simulink model "M1_regOBA_2020b"  (R2020b)
settings: Solver=VariableStepAuto  StartTime=0.0  StopTime=80  RelTol=1e-3
values from neighbouring files (symbols this model uses):
  fsz = 2500    [o01S_model_skryptdrugi.m]
  Jeq = JL + J    (= 3.228252e-05)    [o01S_model_skryptdrugi.m]
  K_windup_p = 1    [o01S_model_skryptdrugi.m]
  K_windup_v = 3    [o01S_model_skryptdrugi.m]
  Km = 0.0257    [o01S_model_skryptdrugi.m]
  Kp_p = 2    [o01S_model_skryptdrugi.m]
  Kp_v = 0.04604    [o01S_model_skryptdrugi.m]
  Psz = 0.005    [o01S_model_skryptdrugi.m]
  Rm = 2.675    [o01S_model_skryptdrugi.m]
  Td_p = 0    [o01S_model_skryptdrugi.m]
  Td_v = 0    [o01S_model_skryptdrugi.m]
  Ti_v = 0.17    [o01S_model_skryptdrugi.m]
  w_filtr_pom = 1/10    (= 0.1)    [o01S_model_skryptdrugi.m]
libraries: simulink x1
settings Model: Creator=Adam  LastModifiedBy=Adam
settings SolverCC: ZeroCrossAlgorithm=Adaptive
settings DebuggingCC: IgnoredZcDiagnostic=none

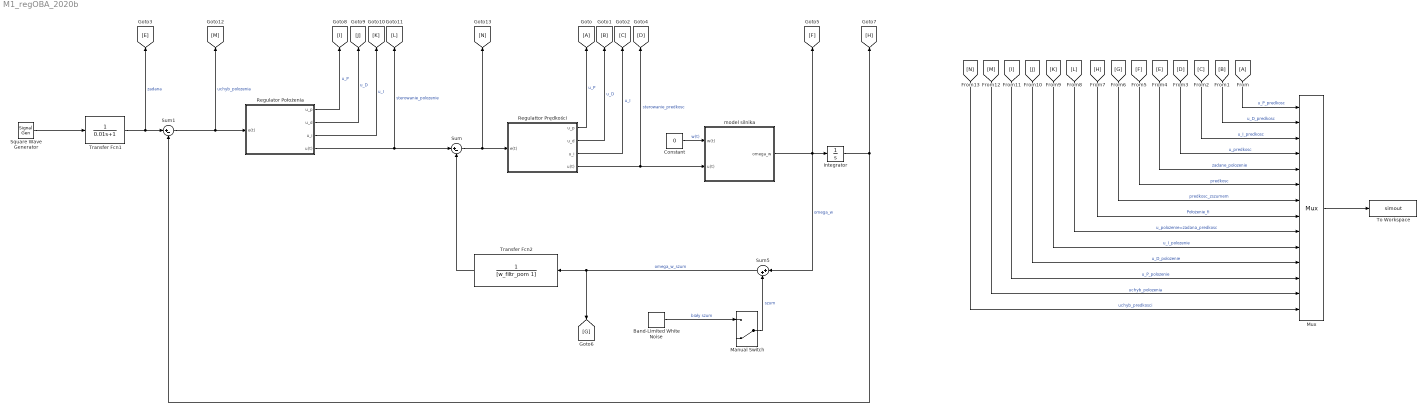
== system M1_regOBA_2020b ==
  Band-Limited White Noise : simulink/Sources/Band-Limited White Noise  Cov=[Psz]  Ts=0.1  seed=[fsz]
  Constant : Constant  Value=0
  Integrator : Integrator
  Manual Switch : ManualSwitch  CurrentSetting=0
  Mux : Mux  Inputs=14
  Regulator Położenia : Subsystem
  Regulattor Prędkości : Subsystem
  Square Wave Generator : SignalGenerator  WaveForm=square  Amplitude=9  Frequency=0.08
  Sum : Sum  Inputs=|+-
  Sum1 : Sum  Inputs=|+-
  Sum5 : Sum  Inputs=|++
  To Workspace : ToWorkspace  VariableName=simout  SaveFormat=Timeseries  SampleTime=-1
  Transfer Fcn1 : TransferFcn  Denominator=[0.01 1]
  Transfer Fcn2 : TransferFcn  Denominator=[w_filtr_pom 1]
  model silnika : Subsystem
  wires:
  Constant/1 -> model silnika/1(w(t))  "w(t)"
  model silnika/1(omega_w) -> Sum5/1, [F], Integrator/1  "omega_w"
  Regulattor Prędkości/4(u(t)) -> model silnika/2(u(t)), [D]  "sterowanie_predkosc"
  Regulattor Prędkości/1(u_p) -> [A]  "u_P"
  Regulattor Prędkości/3(u_i) -> [C]  "u_I"
  Regulattor Prędkości/2(u_d) -> [B]  "u_D"
  Integrator/1 -> [H], Sum1/2
  Manual Switch/1 -> Sum5/2  "szum"
  Sum5/1 -> Transfer Fcn2/1, [G]  "omega_w_szum"
  Band-Limited White Noise/1 -> Manual Switch/1  "biały szum"
  Transfer Fcn2/1 -> Sum/2
  Sum/1 -> Regulattor Prędkości/1(e(t)), [N]
  Square Wave Generator/1 -> Transfer Fcn1/1
  [F] -> Mux/6  "predkosc"
  [A] -> Mux/1  "u_P_predkosc"
  [K] -> Mux/10  "u_I_polozenie"
  [I] -> Mux/12  "u_P_polozenie"
  [N] -> Mux/14  "uchyb_predkosci"
  [G] -> Mux/7  "predkosc_zszumem"
  [M] -> Mux/13  "uchyb_polozenia"
  [L] -> Mux/9  "u_polozenie=zadana_predkosc"
  [J] -> Mux/11  "u_D_polozenie"
  [H] -> Mux/8  "Położenie_fi"
  [B] -> Mux/2  "u_D_predkosc"
  [D] -> Mux/4  "u_predkosc"
  [C] -> Mux/3  "u_I_predkosc"
  [E] -> Mux/5  "zadane_polozenie"
  Mux/1 -> To Workspace/1
  Regulator Położenia/4(u(t)) -> Sum/1, [L]  "sterowanie_polozenie"
  Regulator Położenia/2(u_d) -> [J]  "u_D"
  Regulator Położenia/1(u_p) -> [I]  "u_P"
  Sum1/1 -> [M], Regulator Położenia/1(e(t))  "uchyb_polozenia"
  Regulator Położenia/3(u_i) -> [K]  "u_I"
  Transfer Fcn1/1 -> Sum1/1, [E]  "zadana"

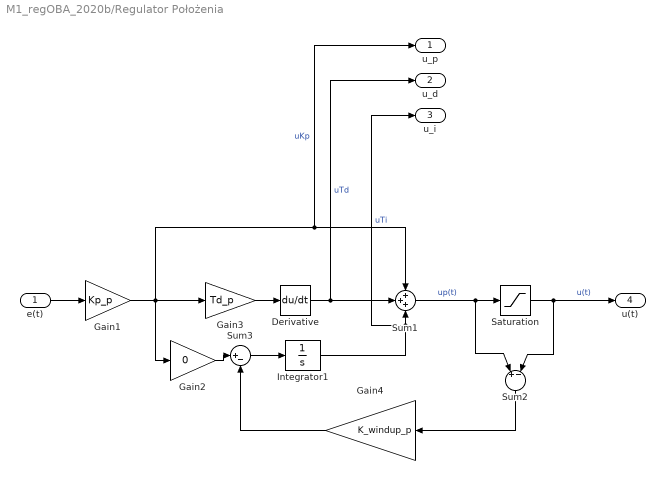
== system M1_regOBA_2020b/Regulator Położenia ==
  e(t) : Inport
  Derivative : Derivative  CoefficientInTFapproximation=500
  Gain1 : Gain  Gain=Kp_p
  Gain2 : Gain  Gain=0
  Gain3 : Gain  Gain=Td_p
  Gain4 : Gain  Gain=K_windup_p
  Integrator1 : Integrator
  Saturation : Saturate  UpperLimit=300  LowerLimit=-300  ZeroCross=off
  Sum1 : Sum  Inputs=+++
  Sum2 : Sum  Inputs=|+-|
  Sum3 : Sum  Inputs=|+-
  u_p : Outport
  u_d : Outport  Port=2
  u_i : Outport  Port=3
  u(t) : Outport  Port=4
  wires:
  Sum1/1 -> Saturation/1, Sum2/1  "up(t)"
  Gain2/1 -> Sum3/1
  Sum2/1 -> Gain4/1
  Gain4/1 -> Sum3/2
  Derivative/1 -> u_d/1, Sum1/2  "uTd"
  Gain3/1 -> Derivative/1
  Gain1/1 -> u_p/1, Sum1/1, Gain3/1, Gain2/1  "uKp"
  Integrator1/1 -> u_i/1, Sum1/3  "uTi"
  Sum3/1 -> Integrator1/1
  Saturation/1 -> u(t)/1, Sum2/2  "u(t)"
  e(t)/1 -> Gain1/1

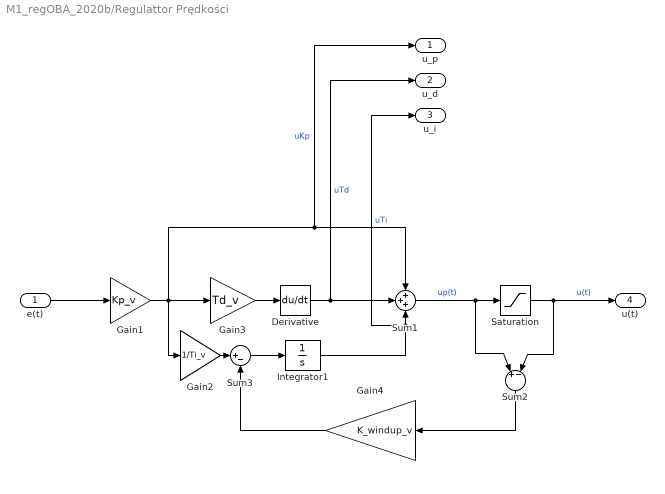
== system M1_regOBA_2020b/Regulattor Prędkości ==
  e(t) : Inport
  Derivative : Derivative  CoefficientInTFapproximation=500
  Gain1 : Gain  Gain=Kp_v
  Gain2 : Gain  Gain=1/Ti_v
  Gain3 : Gain  Gain=Td_v
  Gain4 : Gain  Gain=K_windup_v
  Integrator1 : Integrator
  Saturation : Saturate  UpperLimit=10  LowerLimit=-10  ZeroCross=off
  Sum1 : Sum  Inputs=+++
  Sum2 : Sum  Inputs=|+-|
  Sum3 : Sum  Inputs=|+-
  u_p : Outport
  u_d : Outport  Port=2
  u_i : Outport  Port=3
  u(t) : Outport  Port=4
  wires:
  Sum1/1 -> Saturation/1, Sum2/1  "up(t)"
  Gain2/1 -> Sum3/1
  Sum2/1 -> Gain4/1
  Gain4/1 -> Sum3/2
  Derivative/1 -> u_d/1, Sum1/2  "uTd"
  Gain3/1 -> Derivative/1
  Gain1/1 -> u_p/1, Sum1/1, Gain3/1, Gain2/1  "uKp"
  Integrator1/1 -> u_i/1, Sum1/3  "uTi"
  Sum3/1 -> Integrator1/1
  Saturation/1 -> u(t)/1, Sum2/2  "u(t)"
  e(t)/1 -> Gain1/1

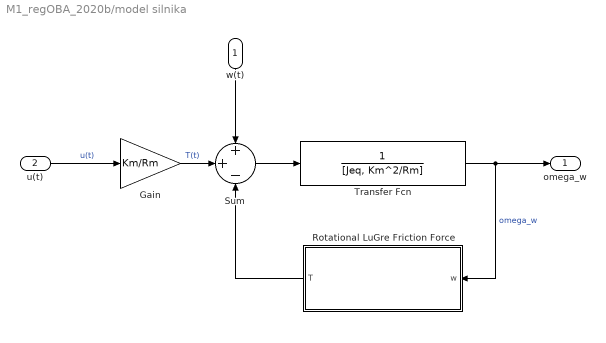
== system M1_regOBA_2020b/model silnika ==
  w(t) : Inport
  u(t) : Inport  Port=2
  Gain : Gain  Gain=Km/Rm
  Rotational LuGre Friction Force : Subsystem  TreatAsAtomicUnit=on  mask(LuGre friction model){ro0=1.2, ro1=0.05, ro2=2.9e-6, Fc=0.77e-3, Fs=12e-3, Vs=0.09}
      mask prompts: Fc "Culomb force (Fc)"; Fs "Friction force (Fs)"; Vs "Striback velocity (Vs)"
      mask help:
      | The LuGre model is a dynamic friction model. The model is related to the bristle interpretation of friction. Friction is modeled as the average deflection force of elastic springs. When a tangential force is applied the bristles will deflect like springs. If the deflection is sufficiently large the bristles start to slip.
      |
      | The input signal is the velocity of the object. The output signal is the fristion force value.
      mask Help:
      | <!DOCTYPE html   PUBLIC "-//W3C//DTD HTML 4.01 Transitional//EN" "http://www.w3.org/TR/1999/REC-html401-19991224/loose.dtd">
      | <html lang="en"><head>
      | <meta http-equiv="Content-Type" content="text/html; charset=utf-8">
      | <title>About :: LuGre friction model</title>
      | <meta name="description" content="">
      | </head>
      | <body><a name="top_of_page"></a>
      | The LuGre model is a dynamic friction model. The model is related to
      | the bristle interpretation of friction. Friction is modeled as the average
      | deflection force of elastic springs. When a tangential force is applied the bristles
      | will deflect like springs. If the deflection is sufficiently large the bristles start
      | to slip. The average bristle deflection for a steady state motion is determined
      | by the velocity. It is lower at low velocities, which implies that the steady state
      | deflection decreases with increasing velocity. This models the phenomenon that
      | the surfaces are pushed apart by the lubricant, and models the Stribeck effect.
      | The model also includes rate dependent friction phenomena such as varying
      | break-away force and frictional lag.<sup><a href="#ref1">1</a></sup></p><p>More information about the model may be found in the labsheets.</p>
      | <hr><small>
      | <sup><a name="ref1"></a>1</sup> <b>Friction Models and Friction Compensation</b>. H. Olsson, K.J. &Aring;str&ouml;m, C. Canudas de Wit, M. G&auml;fvert, P. Lischinsky
      | </small>
      | <br />
      | <br />
      | <hr>
      | <center><small>Copyright&copy;2009
      | <a href="mailto:w.kurek@ely.pg.gda.pl">Wojciech Kurek</a>,
      | <a href="mailto:g.ewald@ely.pg.gda.pl">Grzegorz Ewald</a>
      | </small></center>
      | </body>
      | </html>
      mask Callback ro0:
      | if str2num(get_param(gcb, 'ro0')) <= 0
      |     error('ro0 is negative!')
      | end
      mask Callback ro1:
      | if str2num(get_param(gcb, 'ro1')) <= 0
      |     error('ro1 is negative!')
      | end
      mask Callback ro2:
      | if str2num(get_param(gcb, 'ro2')) <= 0
      |     error('ro2 is negative!')
      | end
      mask Callback Fc:
      | if str2num(get_param(gcb, 'Fs')) <= 0
      |     error('Culomb force is negative!')
      | end
      mask Callback Fs:
      | if str2num(get_param(gcb, 'Fs')) <= 0
      |     error('Friction force is negative!')
      | end
      mask Callback Vs:
      | if str2num(get_param(gcb, 'Vs')) <= 0
      |     error('Striback velocity is negative!')
      | end
      mask Display:
      | patch([0.1 0.1 0.9 0.9],[0.1 0.25 0.25 0.1],[0.8 0.8 0.8])
      | patch([0.1 0.1 0.9 0.9],[0.9 0.75 0.75 0.9],[0.8 0.8 0.8])
      | 
      | plot([0.12 0.12],[0.25 0.5])
      | plot([0.2 0.2],[0.25 0.5])
      | plot([0.4 0.4],[0.25 0.5])
      | plot([0.57 0.57],[0.25 0.5])
      | plot([0.67 0.67],[0.25 0.5])
      | plot([0.87 0.87],[0.25 0.5])
      | 
      | plot([0.17 0.18 0.2 0.23],[0.75 0.6 0.5 0.45])
      | plot([0.35 0.36 0.39 0.44],[0.75 0.6 0.5 0.48])
      | plot([0.62 0.64 0.68 0.72],[0.75 0.6 0.5 0.48])
      | plot([0.85 0.86 0.87 0.89],[0.75 0.6 0.5 0.48])
      | 
      | plot([0.15 0.15],[0.75 0.4])
      | plot([0.28 0.28],[0.75 0.4])
      | plot([0.55 0.55],[0.75 0.4])
      | plot([0.8 0.8],[0.75 0.4])
      | 
      | color('blue');
      | port_label('input',1,'\omega','texmode','on')
      | port_label('output',1,'T','texmode','on')
  Sum : Sum  Inputs=++-
  Transfer Fcn : TransferFcn  Denominator=[Jeq, Km^2/Rm]
  omega_w : Outport
  wires:
  Transfer Fcn/1 -> Rotational LuGre Friction Force/1(w), omega_w/1  "omega_w"
  Rotational LuGre Friction Force/1(T) -> Sum/3
  w(t)/1 -> Sum/1
  Sum/1 -> Transfer Fcn/1
  Gain/1 -> Sum/2  "T(t)"
  u(t)/1 -> Gain/1  "u(t)"

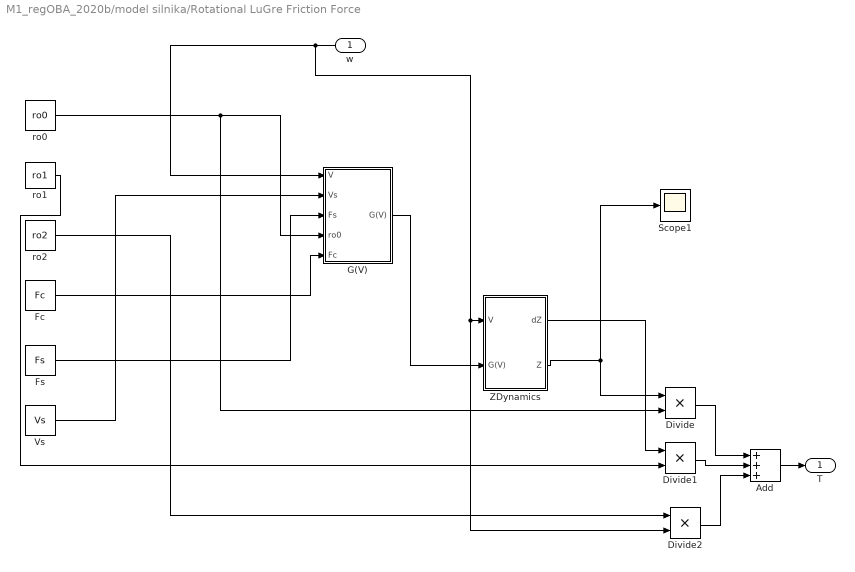
== system M1_regOBA_2020b/model silnika/Rotational LuGre Friction Force ==
  w : Inport
  Add : Sum  Inputs=+++
  Divide : Product  Inputs=**
  Divide1 : Product  Inputs=**
  Divide2 : Product  Inputs=**
  Fc : Constant  Value=Fc
  Fs : Constant  Value=Fs
  G(V) : Subsystem
  Scope1 : Scope
  Vs : Constant  Value=Vs
  ZDynamics : Subsystem
  ro0 : Constant  Value=ro0
  ro1 : Constant  Value=ro1
  ro2 : Constant  Value=ro2
  T : Outport
  wires:
  Add/1 -> T/1
  Divide2/1 -> Add/3
  Divide1/1 -> Add/2
  Divide/1 -> Add/1
  ro2/1 -> Divide2/1
  ro1/1 -> Divide1/2
  ZDynamics/1(dZ) -> Divide1/1
  ZDynamics/2(Z) -> Scope1/1, Divide/1
  G(V)/1(G(V)) -> ZDynamics/2(G(V))
  ro0/1 -> Divide/2, G(V)/4(ro0)
  Fc/1 -> G(V)/5(Fc)
  Fs/1 -> G(V)/3(Fs)
  Vs/1 -> G(V)/2(Vs)
  w/1 -> G(V)/1(V), ZDynamics/1(V), Divide2/2

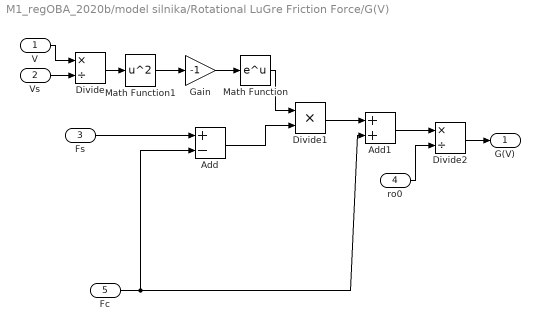
== system M1_regOBA_2020b/model silnika/Rotational LuGre Friction Force/G(V) ==
  V : Inport
  Vs : Inport  Port=2
  Fs : Inport  Port=3
  ro0 : Inport  Port=4
  Fc : Inport  Port=5
  Add : Sum  Inputs=+-
  Add1 : Sum
  Divide : Product  Inputs=*/
  Divide1 : Product  Inputs=**
  Divide2 : Product  Inputs=*/
  Gain : Gain  Gain=-1
  Math Function : Math  SignedPower=on  SaturateOnIntegerOverflow=on
  Math Function1 : Math  Operator=square  SignedPower=on  SaturateOnIntegerOverflow=on
  G(V) : Outport
  wires:
  Math Function/1 -> Divide1/1
  Gain/1 -> Math Function/1
  Math Function1/1 -> Gain/1
  ro0/1 -> Divide2/2
  Divide2/1 -> G(V)/1
  Fs/1 -> Add/1
  Vs/1 -> Divide/2
  V/1 -> Divide/1
  Add1/1 -> Divide2/1
  Divide1/1 -> Add1/1
  Add/1 -> Divide1/2
  Fc/1 -> Add/2, Add1/2
  Divide/1 -> Math Function1/1

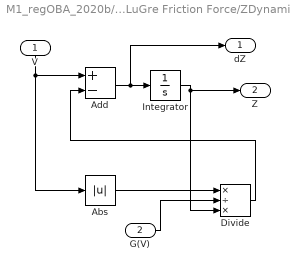
== system M1_regOBA_2020b/model silnika/Rotational LuGre Friction Force/ZDynamics ==
  V : Inport
  G(V) : Inport  Port=2
  Abs : Abs
  Add : Sum  Inputs=+-
  Divide : Product  Inputs=*/*
  Integrator : Integrator
  dZ : Outport
  Z : Outport  Port=2
  wires:
  G(V)/1 -> Divide/2
  V/1 -> Abs/1, Add/1
  Divide/1 -> Add/2
  Integrator/1 -> Z/1, Divide/3
  Abs/1 -> Divide/1
  Add/1 -> dZ/1, Integrator/1
